simulink model "sampleModel1736"  (R2023a)
settings: Solver=VariableStepAuto  StartTime=0.0  StopTime=10.0  RelTol=1e-3
libraries: hdlsllib x4, simulink x2
settings Model: Creator=user1  LastModifiedBy=user1

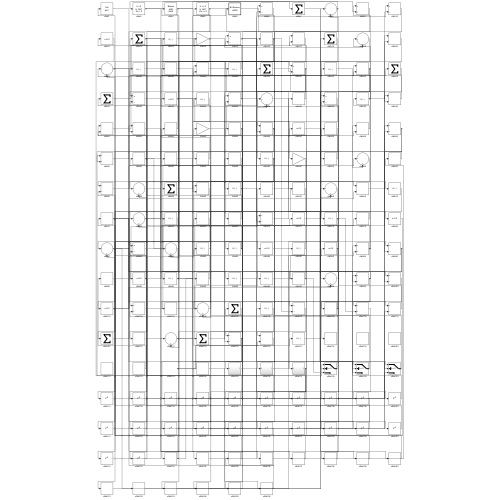
[thumbnail: Simulink's stored preview of the top-level diagram]
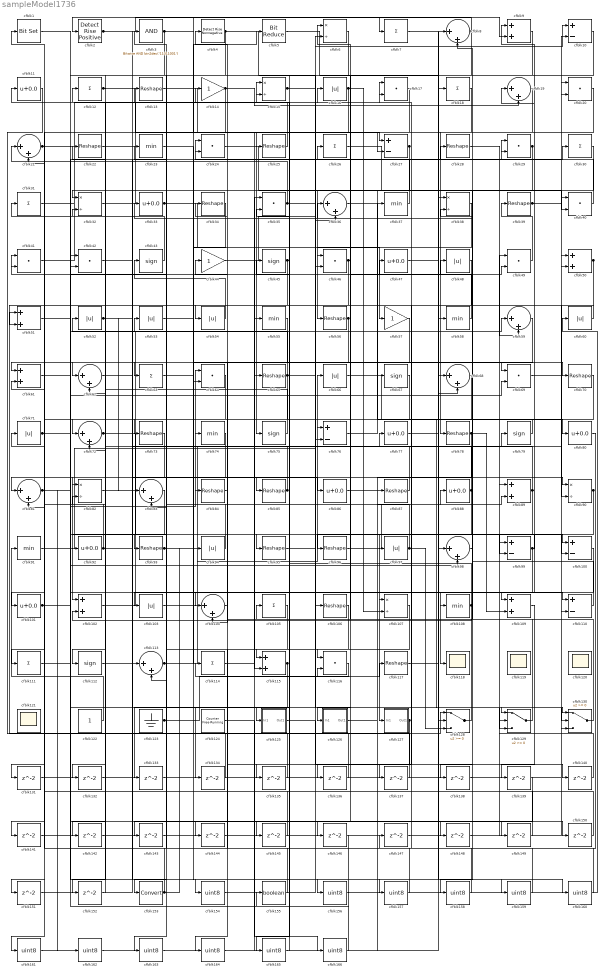
== system sampleModel1736 ==
  cfblk1 : simulink/Logic and Bit Operations/Bit Set  iBit=0
      settings: LibrarySourceBlock=|
      | hdlsllib/Logic and Bit
      | Operations/Bit Set
  cfblk{10,27,76,99..100,110} (6 alike) : Sum  Inputs=+-
  cfblk{11,33,47,77,80,86,88,92,101} (9 alike) : Bias  Bias=0.0  SaturateOnIntegerOverflow=off
  cfblk{9,50..51,61,89,102,109,115} (8 alike) : Sum
  cfblk{16,48,52..54,60,66,71,94,97,103} (11 alike) : Abs  SaturateOnIntegerOverflow=off
  cfblk{8,19,21,36,59,62,68,72,81,83,98,104,113} (13 alike) : Sum  Inputs=|++
  cfblk{7,12,18,26,30..31,63,105,111,114} (10 alike) : Sum  Inputs=+
  cfblk{13,22,25,28,34,39,56,65,70,73,78,84..85,87,93,95..96,106,117} (19 alike) : Reshape
  cfblk{6,15,32,38,82,90,107} (7 alike) : Product  Inputs=*/  RndMeth=Zero  SaturateOnIntegerOverflow=on
  cfblk{23,37,55,58,74,91,108} (7 alike) : MinMax
  cfblk{43,45,67,75,79,112} (6 alike) : Signum
  cfblk{17,20,24,29,35,40..42,46,49,64,69,116} (13 alike) : DotProduct  OutDataTypeStr=Inherit: Inherit via internal rule
  cfblk{118..121} (4 alike) : Scope
      cfblk119 settings: Floating=on
      cfblk120 settings: Floating=on
      cfblk121 settings: Floating=on
  cfblk122 : Constant  SampleTime=-1
  cfblk123 : Ground
  cfblk124 : hdlsllib/Sources/Counter Free-Running  NumBits=16  tsamp=-1
  cfblk125 : Subsystem
      settings: LibrarySourceBlock=|
      | hdlsllib/Ports &
      | Subsystems/Subsystem
  cfblk126 : Subsystem
      settings: LibrarySourceBlock=|
      | hdlsllib/Ports &
      | Subsystems/Subsystem
  cfblk127 : Subsystem
      settings: LibrarySourceBlock=|
      | hdlsllib/Ports &
      | Subsystems/Subsystem
  cfblk128 : Switch  SaturateOnIntegerOverflow=off  InputSameDT=off
  cfblk129 : Switch  SaturateOnIntegerOverflow=off  InputSameDT=off
  cfblk130 : Switch  SaturateOnIntegerOverflow=off  InputSameDT=off
  cfblk{131..152} (22 alike) : Delay  SampleTime=1
  cfblk14 : Gain
  cfblk153 : DataTypeConversion  SaturateOnIntegerOverflow=off  RndMeth=Floor
  cfblk{154,156..166} (12 alike) : DataTypeConversion  OutDataTypeStr=uint8  SaturateOnIntegerOverflow=off  RndMeth=Floor
  cfblk155 : DataTypeConversion  OutDataTypeStr=boolean  SaturateOnIntegerOverflow=off  RndMeth=Floor
  cfblk2 : hdlsllib/Logic and Bit Operations/Detect Rise Positive  vinit=0  OutDataTypeStr=boolean
  cfblk3 : simulink/Logic and Bit Operations/Bitwise Operator  logicop=AND  UseBitMask=on  BitMask=bin2dec('11011001')  BitMaskRealWorld=Stored Integer
      settings: LibrarySourceBlock=|
      | hdlsllib/Logic and Bit
      | Operations/Bitwise
      | Operator
  cfblk4 : hdlsllib/Logic and Bit Operations/Detect Rise Nonnegative  vinit=0  OutDataTypeStr=boolean
  cfblk44 : Gain
  cfblk5 : hdlsllib/Logic and Bit Operations/Bit Reduce  mode=AND
  cfblk57 : Gain
  wires:
  cfblk103/1 -> cfblk77/1
  cfblk20/1 -> cfblk78/1
  cfblk106/1 -> cfblk153/1
  cfblk35/1 -> cfblk21/1, cfblk28/1
  cfblk122/1 -> cfblk91/1
  cfblk104/1 -> cfblk44/1
  cfblk66/1 -> cfblk130/1
  cfblk97/1 -> cfblk64/1, cfblk128/3
  cfblk33/1 -> cfblk57/1, cfblk46/2
  cfblk76/1 -> cfblk37/1
  cfblk17/1 -> cfblk75/1
  cfblk8/1 -> cfblk2/1, cfblk46/1
  cfblk29/1 -> cfblk56/1, cfblk128/2
  cfblk114/1 -> cfblk55/1
  cfblk72/1 -> cfblk100/1, cfblk49/2
  cfblk88/1 -> cfblk127/1(In1), cfblk17/2, cfblk146/1
  cfblk73/1 -> cfblk111/1
  cfblk100/1 -> cfblk118/1
  cfblk41/1 -> cfblk24/1
  cfblk21/1 -> cfblk17/1, cfblk99/2
  cfblk128/1 -> cfblk36/1
  cfblk59/1 -> cfblk62/1
  cfblk77/1 -> cfblk38/1
  cfblk113/1 -> cfblk66/1, cfblk5/1
  cfblk93/1 -> cfblk79/1, cfblk23/1, cfblk129/1
  cfblk54/1 -> cfblk43/1
  cfblk30/1 -> cfblk108/1
  cfblk99/1 -> cfblk19/1, cfblk158/1
  cfblk40/1 -> cfblk4/1
  cfblk70/1 -> cfblk72/1
  cfblk36/1 -> cfblk80/1
  cfblk32/1 -> cfblk16/1
  cfblk13/1 -> cfblk65/1
  cfblk34/1 -> cfblk64/2
  cfblk56/1 -> cfblk112/1, cfblk104/2
  cfblk63/1 -> cfblk70/1
  cfblk52/1 -> cfblk30/1, cfblk83/1
  cfblk82/1 -> cfblk18/1
  cfblk11/1 -> cfblk128/1
  cfblk31/1 -> cfblk15/1
  cfblk24/1 -> cfblk67/1
  cfblk84/1 -> cfblk14/1
  cfblk12/1 -> cfblk25/1, cfblk92/1, cfblk86/1
  cfblk74/1 -> cfblk102/1
  cfblk4/1 -> cfblk63/1, cfblk76/2
  cfblk90/1 -> cfblk109/1, cfblk138/1
  cfblk116/1 -> cfblk114/1
  cfblk107/1 -> cfblk116/1
  cfblk60/1 -> cfblk54/1
  cfblk86/1 -> cfblk90/1
  cfblk81/1 -> cfblk129/3, cfblk69/2, cfblk162/1
  cfblk110/1 -> cfblk33/1
  cfblk75/1 -> cfblk22/1
  cfblk115/1 -> cfblk133/1, cfblk134/1
  cfblk10/1 -> cfblk96/1
  cfblk49/1 -> cfblk39/1
  cfblk79/1 -> cfblk73/1
  cfblk89/1 -> cfblk29/1, cfblk76/1, cfblk148/1
  cfblk102/1 -> cfblk50/2
  cfblk2/1 -> cfblk9/2, cfblk154/1
  cfblk48/1 -> cfblk51/2
  cfblk98/1 -> cfblk38/2
  cfblk9/1 -> cfblk85/1
  cfblk5/1 -> cfblk98/1
  cfblk85/1 -> cfblk81/1, cfblk41/2
  cfblk22/1 -> cfblk27/1
  cfblk14/1 -> cfblk32/1, cfblk19/2
  cfblk26/1 -> cfblk58/1
  cfblk25/1 -> cfblk11/1
  cfblk129/1 -> cfblk52/1
  cfblk94/1 -> cfblk41/1
  cfblk7/1 -> cfblk100/2
  cfblk108/1 -> cfblk103/1, cfblk102/2, cfblk45/1
  cfblk87/1 -> cfblk13/1
  cfblk96/1 -> cfblk88/1
  cfblk46/1 -> cfblk126/1(In1), cfblk115/1
  cfblk91/1 -> cfblk36/2
  cfblk44/1 -> cfblk10/1
  cfblk101/1 -> cfblk84/1, cfblk98/2
  cfblk27/1 -> cfblk115/2, cfblk132/1
  cfblk57/1 -> cfblk61/1
  cfblk58/1 -> cfblk6/1
  cfblk50/1 -> cfblk90/2, cfblk137/1
  cfblk51/1 -> cfblk26/1
  cfblk37/1 -> cfblk24/2
  cfblk117/1 -> cfblk130/2
  cfblk16/1 -> cfblk113/2, cfblk83/2, cfblk107/2
  cfblk43/1 -> cfblk31/1
  cfblk55/1 -> cfblk93/1
  cfblk62/1 -> cfblk95/1
  cfblk112/1 -> cfblk74/1
  cfblk71/1 -> cfblk107/1, cfblk97/1, cfblk150/1
  cfblk45/1 -> cfblk125/1(In1), cfblk141/1
  cfblk126/1(Out1) -> cfblk89/2
  cfblk65/1 -> cfblk129/2, cfblk3/1, cfblk104/1, cfblk135/1
  cfblk111/1 -> cfblk59/1
  cfblk92/1 -> cfblk29/2, cfblk61/2, cfblk152/1
  cfblk123/1 -> cfblk117/1, cfblk116/2
  cfblk130/1 -> cfblk8/2
  cfblk3/1 -> cfblk42/2, cfblk27/2, cfblk7/1
  cfblk95/1 -> cfblk110/1
  cfblk69/1 -> cfblk10/2
  cfblk127/1(Out1) -> cfblk144/1, cfblk145/1
  cfblk28/1 -> cfblk59/2
  cfblk6/1 -> cfblk82/1
  cfblk39/1 -> cfblk20/2, cfblk9/1
  cfblk78/1 -> cfblk101/1, cfblk109/2
  cfblk61/1 -> cfblk48/1
  cfblk15/1 -> cfblk40/2, cfblk69/1
  cfblk67/1 -> cfblk131/1
  cfblk131/1 -> cfblk49/1
  cfblk132/1 -> cfblk40/1
  cfblk133/1 -> cfblk20/1
  cfblk134/1 -> cfblk72/2
  cfblk135/1 -> cfblk32/2
  cfblk38/1 -> cfblk136/1
  cfblk136/1 -> cfblk51/1
  cfblk137/1 -> cfblk15/2
  cfblk138/1 -> cfblk50/1
  cfblk109/1 -> cfblk139/1
  cfblk125/1(Out1) -> cfblk140/1
  cfblk140/1 -> cfblk99/1
  cfblk141/1 -> cfblk110/2
  cfblk83/1 -> cfblk142/1
  cfblk142/1 -> cfblk62/2
  cfblk64/1 -> cfblk143/1
  cfblk143/1 -> cfblk8/1
  cfblk144/1 -> cfblk6/2
  cfblk145/1 -> cfblk82/2
  cfblk80/1 -> cfblk147/1
  cfblk147/1 -> cfblk89/1
  cfblk148/1 -> cfblk130/3
  cfblk23/1 -> cfblk149/1
  cfblk149/1 -> cfblk21/2
  cfblk150/1 -> cfblk35/2
  cfblk19/1 -> cfblk151/1
  cfblk151/1 -> cfblk113/1
  cfblk152/1 -> cfblk12/1
  cfblk153/1 -> cfblk81/2, cfblk94/1
  cfblk154/1 -> cfblk106/1
  cfblk146/1 -> cfblk155/1
  cfblk155/1 -> cfblk1/1
  cfblk1/1 -> cfblk156/1
  cfblk156/1 -> cfblk60/1
  cfblk53/1 -> cfblk157/1
  cfblk157/1 -> cfblk71/1
  cfblk158/1 -> cfblk53/1
  cfblk47/1 -> cfblk159/1
  cfblk159/1 -> cfblk34/1
  cfblk42/1 -> cfblk160/1
  cfblk160/1 -> cfblk47/1
  cfblk68/1 -> cfblk161/1
  cfblk161/1 -> cfblk35/1
  cfblk162/1 -> cfblk68/1
  cfblk139/1 -> cfblk163/1
  cfblk163/1 -> cfblk68/2
  cfblk105/1 -> cfblk164/1
  cfblk164/1 -> cfblk87/1
  cfblk18/1 -> cfblk165/1
  cfblk165/1 -> cfblk105/1
  cfblk124/1 -> cfblk166/1
  cfblk166/1 -> cfblk42/1

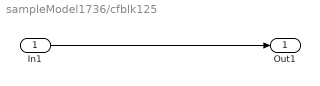
== system sampleModel1736/cfblk125 ==
  In1 : Inport
  Out1 : Outport
  wires:
  In1/1 -> Out1/1

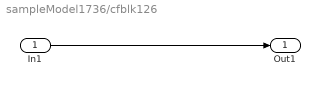
== system sampleModel1736/cfblk126 ==
  In1 : Inport
  Out1 : Outport
  wires:
  In1/1 -> Out1/1

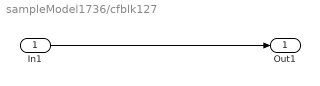
== system sampleModel1736/cfblk127 ==
  In1 : Inport
  Out1 : Outport
  wires:
  In1/1 -> Out1/1
